simulink model "REF_COMPUTATION"  (R2023a)
settings: Solver=VariableStepAuto  StartTime=0.0  StopTime=25  RelTol=1e-3
values from neighbouring files (symbols this model uses):
  Ts = 0.001    [TRAJ.m]
settings Model: Creator=39388  LastModifiedBy=39388

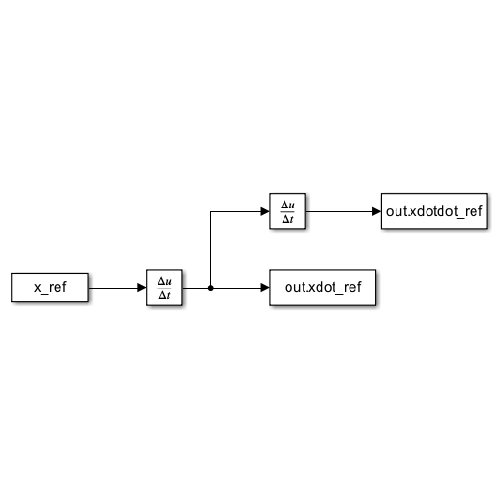
[thumbnail: Simulink's stored preview of the top-level diagram]
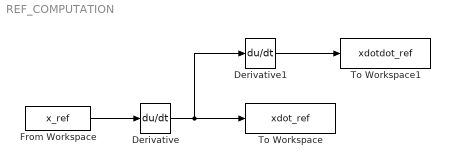
== system REF_COMPUTATION ==
  Derivative : Derivative
  Derivative1 : Derivative
  From Workspace : FromWorkspace  VariableName=x_ref  SampleTime=Ts
  To Workspace : ToWorkspace  VariableName=xdot_ref  SaveFormat=Structure With Time  SampleTime=Ts
  To Workspace1 : ToWorkspace  VariableName=xdotdot_ref  SaveFormat=Structure With Time  SampleTime=Ts
  wires:
  From Workspace/1 -> Derivative/1
  Derivative/1 -> Derivative1/1, To Workspace/1
  Derivative1/1 -> To Workspace1/1
